simulink model "model4_RobustTracking"  (R2020a)
settings: Solver=FixedStepAuto  StartTime=0.0  StopTime=T  FixedStep=Ts  RelTol=1e-3
undefined symbols (not defined in the file): alpha0, alpha1, K, Kz, L, omgn, R, rFlag, stepT, Ts, x0
settings Model: Creator=XiaoCY  LastModifiedBy=XiaoCY
settings DataIOCC: ReturnWorkspaceOutputs=off

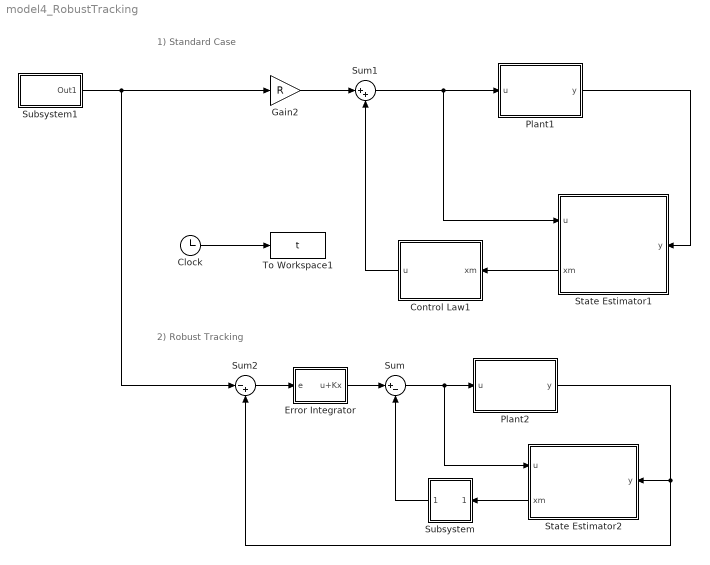
== system model4_RobustTracking ==
  note: 1) Standard Case
  note: 2) Robust Tracking
  Clock : Clock
  Control Law1 : Subsystem
  Error Integrator : Subsystem
  Gain2 : Gain  Gain=R
  Plant1 : Subsystem
  Plant2 : Subsystem
  State Estimator1 : Subsystem
      settings: PortSchema="{\"entries\":[{\"content\":{\"sides\":[{\"content\":{\"connectorIds\":[\"In1\"]},\"type\":\"ConnectorPlacement.EquallySpacedRectSide\",\"uuid\":\"995efd48-3db5-4a6e-85f6-a349d6a63930\"},{\"content\":{\"connectorIds\":[\"In2\",\"Out1\"],\"side\":\"RIGHT\"},\"type\":\"ConnectorPlacement.EquallySpacedRectSide\",\"uuid\":\"626e22d4-5752-4239-b2ce-472c77ace920\"},{\"content\":{\"connectorIds\":[],\"side\":\"TOP\"},\"type\":\"ConnectorPlacement.EquallySpacedRectSide\",\"uuid\":\"cb599412-420c-4014-940e-49f432b7cbea\"}]},\"type\":\"ConnectorPlacement.EquallySpacedConnector\",\"uuid\":\"e0cccee1-86a0-41f4-a3e5-9044b1b28e69\"}],\"packageUris\":[\"http://schema.mathworks.com/mf0/Connector/19700101\"],\"version\":\"1.0\"}"
  State Estimator2 : Subsystem
      settings: PortSchema="{\"entries\":[{\"content\":{\"sides\":[{\"content\":{\"connectorIds\":[\"In1\"]},\"type\":\"ConnectorPlacement.EquallySpacedRectSide\",\"uuid\":\"995efd48-3db5-4a6e-85f6-a349d6a63930\"},{\"content\":{\"connectorIds\":[\"In2\",\"Out1\"],\"side\":\"RIGHT\"},\"type\":\"ConnectorPlacement.EquallySpacedRectSide\",\"uuid\":\"626e22d4-5752-4239-b2ce-472c77ace920\"},{\"content\":{\"connectorIds\":[],\"side\":\"TOP\"},\"type\":\"ConnectorPlacement.EquallySpacedRectSide\",\"uuid\":\"cb599412-420c-4014-940e-49f432b7cbea\"}]},\"type\":\"ConnectorPlacement.EquallySpacedConnector\",\"uuid\":\"e0cccee1-86a0-41f4-a3e5-9044b1b28e69\"}],\"packageUris\":[\"http://schema.mathworks.com/mf0/Connector/19700101\"],\"version\":\"1.0\"}"
  Subsystem : Subsystem
      mask Display: disp('Kx')
  Subsystem1 : Subsystem
      mask Display: disp('Reference')
  Sum : Sum  Inputs=|+-
  Sum1 : Sum  Inputs=|++
  Sum2 : Sum  Inputs=|-+
  To Workspace1 : ToWorkspace  VariableName=t  SampleTime=Ts
  wires:
  Clock/1 -> To Workspace1/1
  Gain2/1 -> Sum1/1
  Sum1/1 -> State Estimator1/2(u), Plant1/1(u)
  Control Law1/1(u) -> Sum1/2
  State Estimator1/1(xm) -> Control Law1/1(xm)
  Plant1/1(y) -> State Estimator1/1(y)
  Sum/1 -> State Estimator2/2(u), Plant2/1(u)
  Plant2/1(y) -> State Estimator2/1(y), Sum2/2
  Sum2/1 -> Error Integrator/1(e)
  Error Integrator/1(u+Kx) -> Sum/1
  State Estimator2/1(xm) -> Subsystem/1(In1)
  Subsystem/1(Out1) -> Sum/2
  Subsystem1/1(Out1) -> Sum2/1, Gain2/1

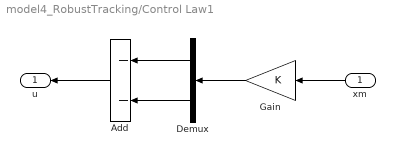
== system model4_RobustTracking/Control Law1 ==
  xm : Inport
  Add : Sum  Inputs=--
  Demux : Demux  Outputs=2
  Gain : Gain  Gain=K
  u : Outport
  wires:
  Demux/1 -> Add/1
  Gain/1 -> Demux/1
  Add/1 -> u/1
  Demux/2 -> Add/2
  xm/1 -> Gain/1

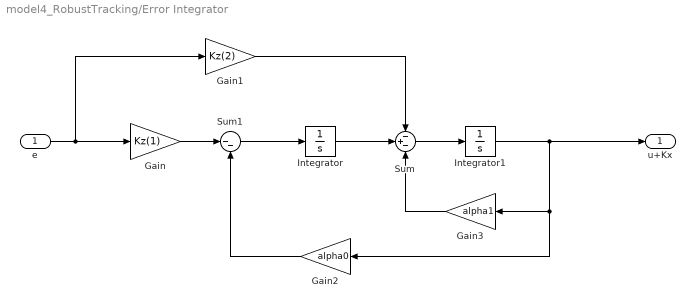
== system model4_RobustTracking/Error Integrator ==
  e : Inport
  Gain : Gain  Gain=Kz(1)
  Gain1 : Gain  Gain=Kz(2)
  Gain2 : Gain  Gain=alpha0
  Gain3 : Gain  Gain=alpha1
  Integrator : Integrator
  Integrator1 : Integrator
  Sum : Sum  Inputs=-+-
  Sum1 : Sum  Inputs=|--
  u+Kx : Outport
  wires:
  Integrator/1 -> Sum/2
  Sum/1 -> Integrator1/1
  e/1 -> Gain1/1, Gain/1
  Sum1/1 -> Integrator/1
  Integrator1/1 -> Gain2/1, Gain3/1, u+Kx/1
  Gain/1 -> Sum1/1
  Gain1/1 -> Sum/1
  Gain3/1 -> Sum/3
  Gain2/1 -> Sum1/2

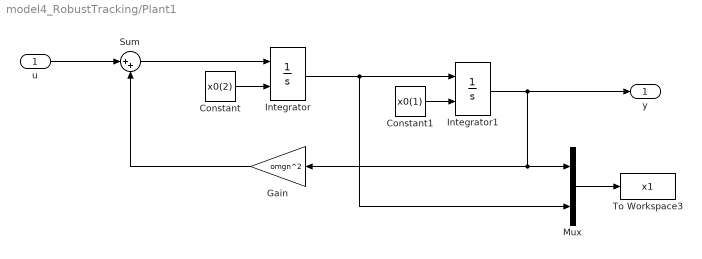
== system model4_RobustTracking/Plant1 ==
  u : Inport
  Constant : Constant  Value=x0(2)
  Constant1 : Constant  Value=x0(1)
  Gain : Gain  Gain=omgn^2
  Integrator : Integrator  InitialConditionSource=external
  Integrator1 : Integrator  InitialConditionSource=external
  Mux : Mux  Inputs=2
  Sum : Sum  Inputs=|++
  To Workspace3 : ToWorkspace  VariableName=x1  SampleTime=Ts
  y : Outport
  wires:
  Integrator1/1 -> y/1, Mux/1, Gain/1
  Mux/1 -> To Workspace3/1
  Gain/1 -> Sum/2
  Sum/1 -> Integrator/1
  Constant/1 -> Integrator/2
  u/1 -> Sum/1
  Constant1/1 -> Integrator1/2
  Integrator/1 -> Integrator1/1, Mux/2

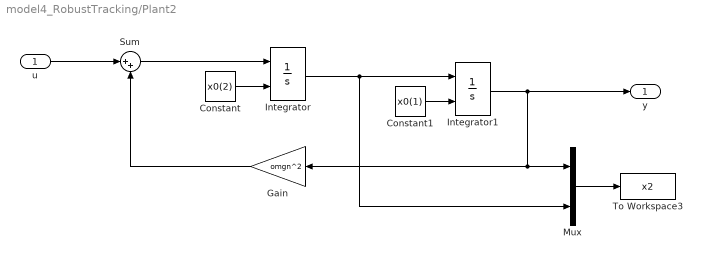
== system model4_RobustTracking/Plant2 ==
  u : Inport
  Constant : Constant  Value=x0(2)
  Constant1 : Constant  Value=x0(1)
  Gain : Gain  Gain=omgn^2
  Integrator : Integrator  InitialConditionSource=external
  Integrator1 : Integrator  InitialConditionSource=external
  Mux : Mux  Inputs=2
  Sum : Sum  Inputs=|++
  To Workspace3 : ToWorkspace  VariableName=x2  SampleTime=Ts
  y : Outport
  wires:
  Integrator/1 -> Mux/2, Integrator1/1
  Constant1/1 -> Integrator1/2
  u/1 -> Sum/1
  Constant/1 -> Integrator/2
  Sum/1 -> Integrator/1
  Gain/1 -> Sum/2
  Mux/1 -> To Workspace3/1
  Integrator1/1 -> Gain/1, Mux/1, y/1

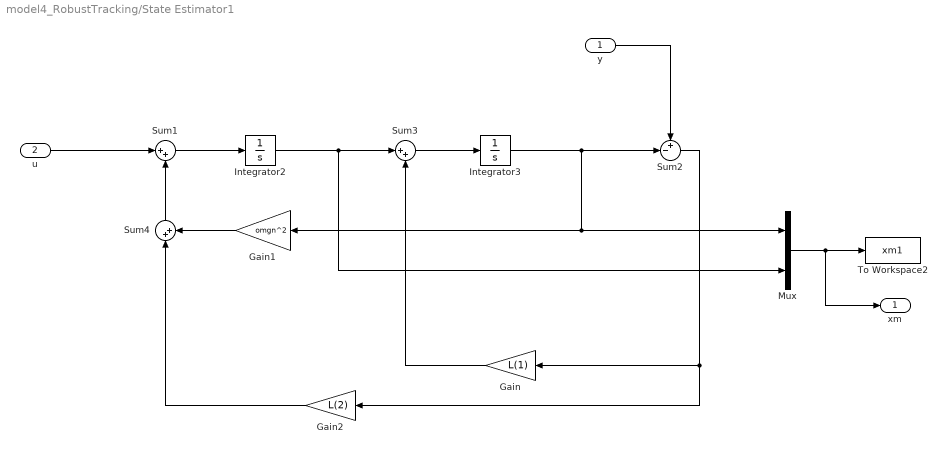
== system model4_RobustTracking/State Estimator1 ==
  y : Inport
  u : Inport  Port=2
  Gain : Gain  Gain=L(1)
  Gain1 : Gain  Gain=omgn^2
  Gain2 : Gain  Gain=L(2)
  Integrator2 : Integrator
  Integrator3 : Integrator
  Mux : Mux  Inputs=2
  Sum1 : Sum  Inputs=|++
  Sum2 : Sum  Inputs=+-|
  Sum3 : Sum  Inputs=|++
  Sum4 : Sum  Inputs=|++
  To Workspace2 : ToWorkspace  VariableName=xm1  SampleTime=Ts
  xm : Outport
  wires:
  Gain2/1 -> Sum4/1
  Gain/1 -> Sum3/2
  Sum4/1 -> Sum1/2
  Gain1/1 -> Sum4/2
  Sum3/1 -> Integrator3/1
  Sum2/1 -> Gain/1, Gain2/1
  Mux/1 -> To Workspace2/1, xm/1
  Integrator2/1 -> Sum3/1, Mux/2
  u/1 -> Sum1/1
  Sum1/1 -> Integrator2/1
  Integrator3/1 -> Gain1/1, Mux/1, Sum2/2
  y/1 -> Sum2/1

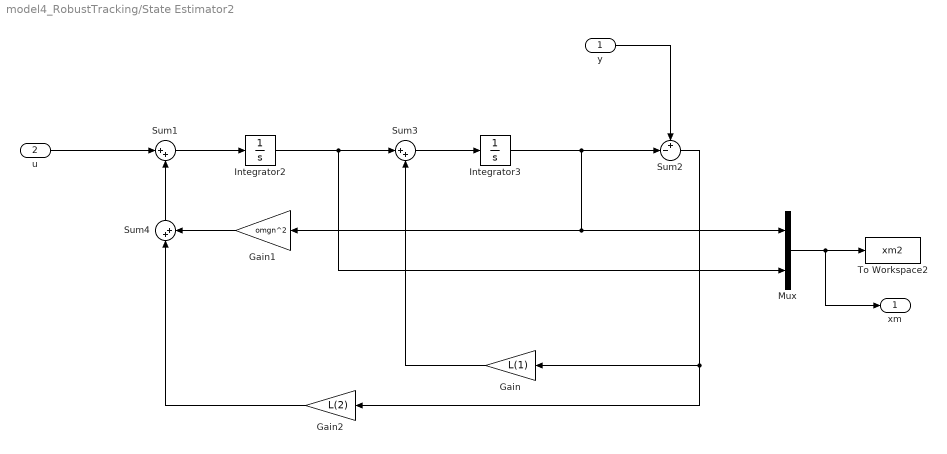
== system model4_RobustTracking/State Estimator2 ==
  y : Inport
  u : Inport  Port=2
  Gain : Gain  Gain=L(1)
  Gain1 : Gain  Gain=omgn^2
  Gain2 : Gain  Gain=L(2)
  Integrator2 : Integrator
  Integrator3 : Integrator
  Mux : Mux  Inputs=2
  Sum1 : Sum  Inputs=|++
  Sum2 : Sum  Inputs=+-|
  Sum3 : Sum  Inputs=|++
  Sum4 : Sum  Inputs=|++
  To Workspace2 : ToWorkspace  VariableName=xm2  SampleTime=Ts
  xm : Outport
  wires:
  y/1 -> Sum2/1
  Integrator3/1 -> Sum2/2, Mux/1, Gain1/1
  Sum1/1 -> Integrator2/1
  u/1 -> Sum1/1
  Integrator2/1 -> Mux/2, Sum3/1
  Mux/1 -> xm/1, To Workspace2/1
  Sum2/1 -> Gain2/1, Gain/1
  Sum3/1 -> Integrator3/1
  Gain1/1 -> Sum4/2
  Sum4/1 -> Sum1/2
  Gain/1 -> Sum3/2
  Gain2/1 -> Sum4/1

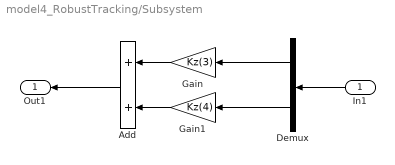
== system model4_RobustTracking/Subsystem ==
  In1 : Inport
  Add : Sum
  Demux : Demux  Outputs=2
  Gain : Gain  Gain=Kz(3)
  Gain1 : Gain  Gain=Kz(4)
  Out1 : Outport
  wires:
  In1/1 -> Demux/1
  Add/1 -> Out1/1
  Gain/1 -> Add/1
  Gain1/1 -> Add/2
  Demux/1 -> Gain/1
  Demux/2 -> Gain1/1

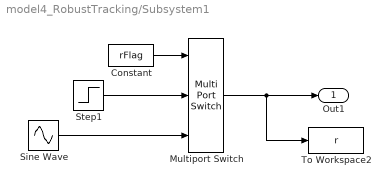
== system model4_RobustTracking/Subsystem1 ==
  Constant : Constant  Value=rFlag
  Multiport Switch : MultiPortSwitch  Inputs=2
  Sine Wave : Sin  Frequency=alpha0  SampleTime=0
  Step1 : Step  Time=stepT  SampleTime=0
  To Workspace2 : ToWorkspace  VariableName=r  SampleTime=Ts
  Out1 : Outport
  wires:
  Sine Wave/1 -> Multiport Switch/3
  Multiport Switch/1 -> To Workspace2/1, Out1/1
  Step1/1 -> Multiport Switch/2
  Constant/1 -> Multiport Switch/1
